simulink model "polydome_python"  (R2020b)
settings: Solver=VariableStepAuto  StartTime=0.0  StopTime=365 * 24 * 3600  RelTol=1e-3
model workspace: external: MAT-File /home/radu/Projects/Master-Project/Simulink/polydome_params.mat (data not in the file)
values from neighbouring files (symbols this model uses):
  Tsample = 900    [model_identification.m]
  window_roof_size = [5 5]    [main.m]
undefined symbols (not defined in the file or in its folder): DE_TRY2010_04_averageYear, Dreifach, f, path_carnot, Wärmeschutzglas
libraries: carnot x13, instrumentlib x3, simulink_extras x2
settings Model: PauseTimes=9200  OrderedModelArguments=off  Creator=radu  LastModifiedBy=radu
settings HardwareCC: ProdBitPerLong=64  ProdHWDeviceType=Intel->x86-64 (Linux 64)

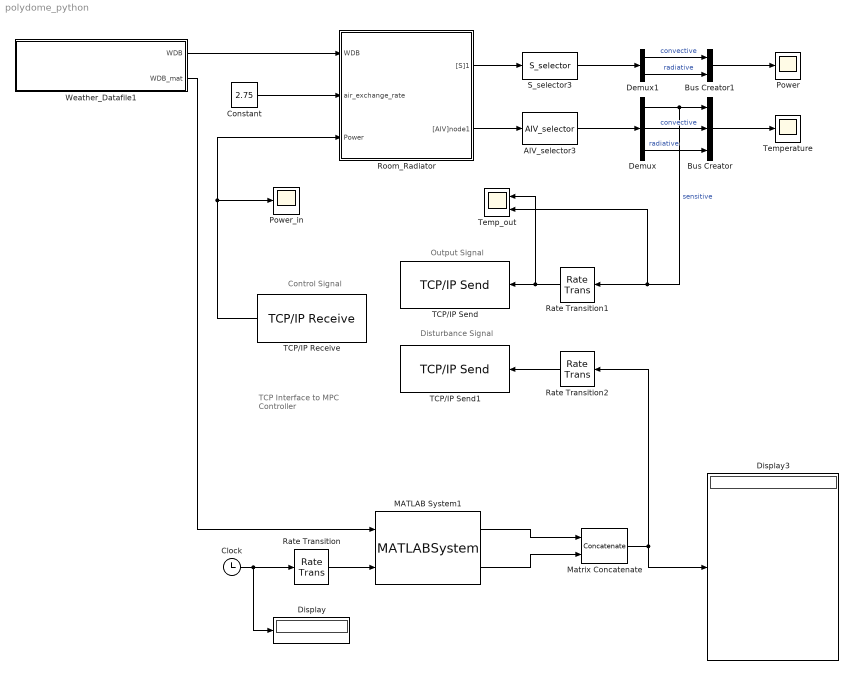
== system polydome_python ==
  note: TCP Interface to
      | MPC Controller
  note: Control Signal
  note: Output Signal
  note: Disturbance Signal
  AIV_selector3 : carnot/Outputs/AIV_selector  e1=on  e2=on  e3=on  e4=off  e5=off  e6=off  e7=off  e8=off  e9=off
      settings: SourceProductName=Carnot
  Bus Creator : BusCreator  Inputs=3
  Bus Creator1 : BusCreator  Inputs=2
  Clock : Clock
  Constant : Constant  Value=2.75
  Demux : Demux  Outputs=3
  Demux1 : Demux  Outputs=2
  Display : Display
  Display3 : Display
  MATLAB System1 : MATLABSystem  System=weather_predictor  TimeStep=Tsample  N=8  SimulateUsing=Interpreted execution
      mask Type: weather_predictor
      mask Display:
      | disp('weather_predictor');
      | port_label('input',1,'wdb_mat');
      | port_label('input',2,'timestamp');
      | port_label('output',1,'w');
      | port_label('output',2,'w_hat');
  Matrix Concatenate : Concatenate  Mode=Multidimensional array
  Power : Scope
  Power_in : Scope
  Rate Transition : RateTransition  OutPortSampleTime=Tsample
  Rate Transition1 : RateTransition  OutPortSampleTime=Tsample
  Rate Transition2 : RateTransition  OutPortSampleTime=Tsample
  Room_Radiator : Subsystem  AncestorBlock=carnot/Load/Houses/Room_Radiator  mask(room){t0=23, temp_neighbour=12}
      mask prompts: t0 "start temperature of rooms in °C"; temp_neighbour "temperature of rooms above and below in °C"
      mask help:
      | The block models of a heat transfer characteristic of two neighbour rooms.
      | Use "look under mask" to set up the models parameters (initial conditions,
      | floors and wall characteristics...)
      mask init:
      | AIV_neighbour = [0 temp_neighbour temp_neighbour 0 0 0 0 0 0];
      | zonefloordist2grnd = 0;
      mask Help: web(fullfile(path_carnot('help'),'Room_Radiator.html'),'-helpbrowser')
      mask Display: plot(0,0,100,100,[30,30,60,60,30],[20,50,50,20,20],[47,47,56,56,47],[40,30,30,40,40],[42,42,34,34],[20,40,40,20],[62,45,28],[48,70,48])
  S_selector3 : carnot/Outputs/S_selector  e1=off  e2=off  e3=off  e4=off  e5=off  e6=off  e7=on  e8=on  e9=off  e10=off  e11=off  e12=off  e13=off
      settings: SourceProductName=Carnot
  TCP/IP Receive : instrumentlib/TCP//IP Receive  Host=127.0.0.1  Port=10001  DataSize=[1 1]  EnableBlockingMode=on  Timeout=100  SampleTime=Tsample  DataType=double  ByteOrder=BigEndian  ASCIIFormatting=%f,  Terminator=LF
  TCP/IP Send : instrumentlib/TCP//IP Send  Host=127.0.0.1  Port=10000  EnableBlockingMode=on  Timeout=10  ByteOrder=BigEndian  TransferDelay=on
  TCP/IP Send1 : instrumentlib/TCP//IP Send  Host=127.0.0.1  Port=10002  EnableBlockingMode=on  Timeout=10  ByteOrder=BigEndian  TransferDelay=on
  Temp_out : Scope  NumInputPorts=2
  Temperature : Scope
  Weather_Datafile1 : Subsystem  AncestorBlock=carnot/Weather/Weather_Datafile  mask(Weather Datafile){PathName=path_carnot('data'), FileName='DE_TRY2010_12_averageYear.mat', UserParam=off, VariableName=DE_TRY2010_04_averageYear, SampleTime=3600}
      mask prompts: PathName "Selected path"; FileName "File"; UserParam "Edit file and path"; VariableName "Simulink:blkprm_prompts:FromWksData"; SampleTime "Timestep in data"
      mask help:
      | Loads weather data in a variable in the mask workspace and extends it according to the simulation interval. A "From Workspace" block in the subsystem uses this variable. The file must contain data in the weather data format of Carnot (type "help WDB_format" in Command window). A Unit-Delay with the timestep of the data forces the model to a maximum timestep equal to the data timestep. This "Timestep in data" is shown as information in the "Selection" frame.
      | Use of buttons in the "Picking a file" frame:
      | 1) "From selected path" opens a window to chose a data file from the "Selected path" shown in the "Selection" frame.
      | 2) "Carnot public data" opens a window to chose a data file from the public data folder in Carnot. The "Path" is set to the public data folder.
      | 3) "Carnot internal data" opens a window to chose a data file from the internal data folder in Carnot. The "Path" is set to the internal data folder.
      | "File" shows the name of the selected file, "Path" the folder where it is located. You can allow editing "File" and "Path" with the checkbox. Be aware that the buttons in the "Picking a file" frame will anyway overwrite the edited values.
      mask init:
      | [ok,VariableName] = CarnotCallbacks_Data_from_File('LoadData', ...
      |     gcbh, PathName, FileName);
      mask Help: web(fullfile(path_carnot('help'),'WeatherDatafile.html'),'-helpbrowser')
      mask Callback UserParam: ok = CarnotCallbacks_Data_from_File('UserMaskEnable',gcbh);
      mask TypeOptions VariableName: FromWorkspace/VariableName
      mask TypeOptions SampleTime: UnitDelay/SampleTime
      mask DialogControl ParameterGroupVar Prompt: Picking a file
      mask DialogControl Control2 Prompt: From selected path
      mask DialogControl Control2 Callback: ok = CarnotCallbacks_Data_from_File('GetFilename',gcbh, 'selected');
      mask DialogControl Control3 Prompt: Carnot public data
      mask DialogControl Control3 Callback: ok = CarnotCallbacks_Data_from_File('GetFilename',gcbh, 'public');
      mask DialogControl Control4 Prompt: Carnot internal data
      mask DialogControl Control4 Callback: ok = CarnotCallbacks_Data_from_File('GetFilename',gcbh, 'internal');
      mask DialogControl Container3 Prompt: Chosen file
      mask DialogControl VariableName Prompt: Data:
      mask Display: disp(['Weather data file:\n', FileName(1:end-4)])
  wires:
  S_selector3/1 -> Demux1/1
  Demux1/1 -> Bus Creator1/1  "convective"
  Demux1/2 -> Bus Creator1/2  "radiative"
  AIV_selector3/1 -> Demux/1
  Room_Radiator/2("[AIV]node1") -> AIV_selector3/1
  Bus Creator1/1 -> Power/1
  Weather_Datafile1/1(WDB) -> Room_Radiator/1(WDB)
  Demux/2 -> Bus Creator/2  "convective"
  Constant/1 -> Room_Radiator/2(air_exchange_rate)
  Demux/3 -> Bus Creator/3  "radiative"
  Bus Creator/1 -> Temperature/1
  Demux/1 -> Bus Creator/1, Temp_out/2, Rate Transition1/1  "sensitive"
  Room_Radiator/1("[S]1") -> S_selector3/1
  Clock/1 -> Rate Transition/1, Display/1
  Weather_Datafile1/2(WDB_mat) -> MATLAB System1/1
  Rate Transition/1 -> MATLAB System1/2
  TCP/IP Receive/1 -> Room_Radiator/3(Power), Power_in/1
  Rate Transition1/1 -> Temp_out/1, TCP/IP Send/1
  Rate Transition2/1 -> TCP/IP Send1/1
  MATLAB System1/1 -> Matrix Concatenate/1
  MATLAB System1/2 -> Matrix Concatenate/2
  Matrix Concatenate/1 -> Rate Transition2/1, Display3/1

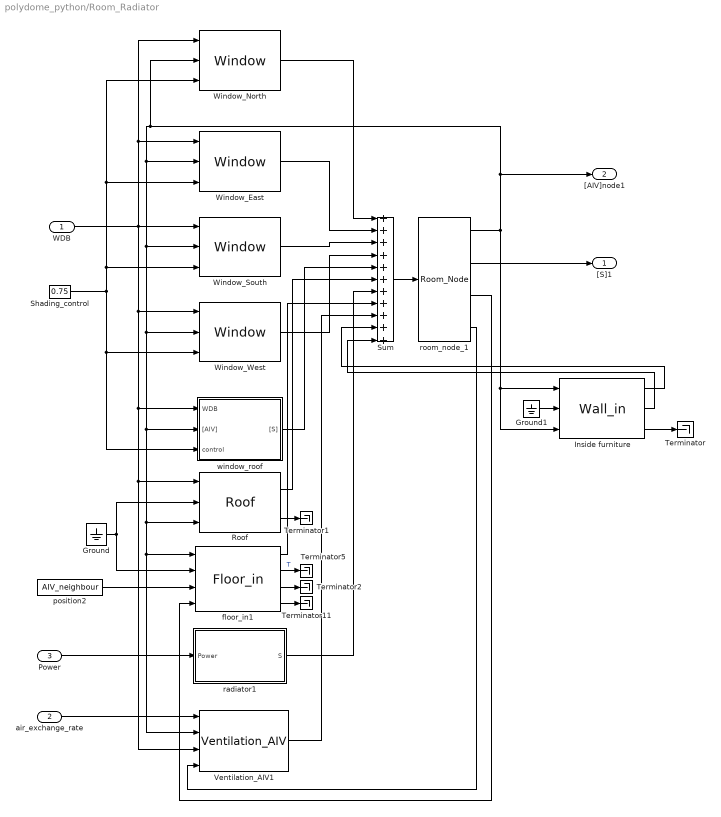
== system polydome_python/Room_Radiator ==
  WDB : Inport
  air_exchange_rate : Inport  Port=2
  Power : Inport  Port=3
  Ground : Ground
  Ground1 : Ground
  Inside furniture : carnot/Basic/Thermal_Models/Wall_in  wallsize=(0.25)*[25 25]*1.8*(1/2)  d=[0.04]  cond=[0.3]  cwall=[1400]  rho=[600]*2  emission_in=.96  dactive=[-1]  t0=t0  tau=10*3600
      settings: SourceProductName=Carnot
  Roof : carnot/Basic/Thermal_Models/Roof  wallsize=wall_size  pos=roof_position  t0=t0  d=node_thickness  cond=node_conductivity  cwall=node_capacity  rho=node_density  reflectground=0.2  abs_emiss=[0.6, 0.9, 0.9]  tau=1000*3600  dactive=-1
      settings: SourceProductName=Carnot
  Shading_control : Constant  Value=0.75
  Sum : Sum  Inputs=11  InputSameDT=on  SaturateOnIntegerOverflow=on  OutDataTypeStr=Inherit: Same as first input
  Terminator{,1..2,5,11} (5 alike) : Terminator
  Ventilation_AIV1 : carnot/Source/Ventilation/Ventilation_AIV  co2=400
      settings: SourceProductName=Carnot
  Window_East : carnot/Basic/Thermal_Models/Window  pos=-80  windowsize=window_size  frame=surface_part  Ug=U  gvalue=g  tauzero=v_g  numpanes=2  d=[0.004 0.004]  rho=[2500 2500]  cp="[1008  1008]"  t0=t0  misc=[0.2 0.1 1 1]  shad_type=Exterior Screen  type_glazing=Dreifach-Wärmeschutzglas  tau_shad=0.01  bli_a=0.05  bli_b=1  bli_c=0.05  bli_d=0.05  bli_alpha=90  bli_refl=0.2
      settings: SourceProductName=Carnot
  Window_North : carnot/Basic/Thermal_Models/Window  pos=-170  windowsize=window_size  frame=surface_part  Ug=U  gvalue=g  tauzero=v_g  numpanes=2  d=[0.004 0.004]  rho=[2500 2500]  cp="[1008  1008]"  t0=t0  misc=[0.2 0.1 1 1]  shad_type=Exterior Screen  type_glazing=Dreifach-Wärmeschutzglas  tau_shad=0.01  bli_a=0.05  bli_b=1  bli_c=0.05  bli_d=0.05  bli_alpha=90  bli_refl=0.2
      settings: SourceProductName=Carnot
  Window_South : carnot/Basic/Thermal_Models/Window  pos=10  windowsize=window_size  frame=surface_part  Ug=U  gvalue=g  tauzero=v_g  numpanes=2  d=[0.004 0.004]  rho=[2500 2500]  cp="[1008  1008]"  t0=t0  misc=[0.2 0.1 1 1]  shad_type=Exterior Screen  type_glazing=Dreifach-Wärmeschutzglas  tau_shad=0.01  bli_a=0.05  bli_b=1  bli_c=0.05  bli_d=0.05  bli_alpha=90  bli_refl=0.2
      settings: SourceProductName=Carnot
  Window_West : carnot/Basic/Thermal_Models/Window  pos=100  windowsize=window_size  frame=surface_part  Ug=U  gvalue=g  tauzero=v_g  numpanes=2  d=[0.004 0.004]  rho=[2500 2500]  cp="[1008  1008]"  t0=t0  misc=[0.2 0.1 1 1]  shad_type=Exterior Screen  type_glazing=Dreifach-Wärmeschutzglas  tau_shad=0.01  bli_a=0.05  bli_b=1  bli_c=0.05  bli_d=0.05  bli_alpha=90  bli_refl=0.2
      settings: SourceProductName=Carnot
  floor_in1 : carnot/Basic/Thermal_Models/Floor_in  wallsize=ceiling_size  t0=t0  d=layer_thickness  cond=layer_conductivity  cwall=layer_capacity  rho=layer_density  misc=[0.9 0.9]  dactive=-1  tau=1000*3600
      settings: SourceProductName=Carnot
  position2 : Constant  Value=AIV_neighbour
  radiator1 : Subsystem  AncestorBlock=carnot/Source/Heat_Exchanger/Radiator_AIV  mask(radiator){pnom=500, dtnom=40, expo=1.3, mcap=5*4182, ra=0.47, tini=24, lin=0, qua=1000}
      mask prompts: pnom "nominal power per unit in W"; dtnom "nominal temperature difference in K"; expo "radiator exponent (> 0)"; mcap "mass * capacity per unit in J/K"; ra "radiative part of heat transfer (0..1)"; tini "initial temperature in degree Celsius"; lin "linear pressure drop dependace of massflow in Pa*s/kg"; qua "quadratic pressure drop dependace of massflow in Pa*s²/kg²"
      mask help: Calculates the power of a radiator according to the nominal power the and the temperaure difference.
      mask init:
      | ra = max(0, min(1, ra));
      | co = 1-ra;
      mask Help: web(['file:///' fullfile(path_carnot('help'),'Radiator.html')],'-helpbrowser')
      mask DialogControl ParameterTabVar0 Prompt: Thermal
      mask DialogControl ParameterTabVar01 Prompt: Hydraulic
      mask Display: plot(-20,0,120,90,[20 90 90 20 20],[20 20 70 70 20],[30 30],[25 65],[40 40],[25 65],[50 50],[25 65],[60 60],[25 65],[70 70],[25 65],[80 80],[25 65],[15 20],[25 25],[15 20],[65 65])
  room_node_1 : carnot/Basic/Thermal_Models/Room_Node  zoneairvolume=25*25*5  zoneheight=2.5  zonestartTEMP=t0  zonestartWATER=55  timeconst=100  heatperfect=natural  lookuptime=[0 24]*3600  lookupvalue=[20 20]  AirPressure=101300  calc_p=off
      settings: SourceProductName=Carnot
  window_roof : Subsystem  AncestorBlock=carnot/Basic/Thermal_Models/Window  mask(window){pos=0, windowsize=window_roof_size, frame=0.1, Ug=1.8, gvalue=0.7, tauzero=0.8, numpanes=2, d=[0.004 0.004], rho=[2500 2500], cp=[1008  1008], t0=t0, misc=[0.2 0.1 1 1], shad_type=No shading, type_glazing=Dreifach-Wärmeschutzglas, tau_shad=0.01, bli_a=0.05, bli_b=1, bli_c=0.05, bli_d=0.05, bli_alpha=90, bli_refl=0.2}
      mask prompts: pos "azimut (0=south, east = -90)"; windowsize "size of window [m] [height width]"; frame "part of frame of the surface (0..1)"; Ug "heat transfer coefficient (U-value) [W/m²K]"; gvalue "total solar energy transmittance (g-value) [0..1]"; tauzero "transmittance in visible range of the sunlight [0..1]"; numpanes "number of glass panes [1..4]"; d "thickness of glass panes [m] (vector with one element per pane)"; rho "density of glass [kg/m³] (vector with one element per pane)"; cp "capacity of glass [J/(kg*K)] (vector with one element per pane)"; t0 "initial temperature [°C]"; misc "[reflection_ground absorption_out emission_out emission_in]"; shad_type "shading type [no Shading/exterior/interior]"; type_glazing "glazing type"; tau_shad "solar transmittance of shading element [0..1]"; bli_a "a  Depth of blind blades [m]"; bli_b "b heigth of blind blades [m]"; bli_c "c distance of "b" to back end of blind blade [m]"; bli_d "d offset between blind blades [m]"; bli_alpha "blind angle  (0=closed, 90=horizontal) [0..90]"; bli_refl "optical reflectance of blind surface [0..1]"
      mask help:
      | The window model evaluates the g-value, the total energy transmission tau and the u-value to build up a two node model.
      | control input [0..1] = fraction of shading (0 - no shading,   1 - full shading)
      mask init:
      | % Geometry
      | h = windowsize(1);
      | w = windowsize(2);
      | windowsurface = h*w;
      | if length(pos) == 1
      |     pos = [0  pos 0]; % pos is [inclination azimut rotation]
      | end
      | 
      | % Optics
      | reflectground = max(0, min(1, misc(1)));
      | absorption_out = max(0, min(1, misc(2)));
      | emission_out = max(0, min(1, misc(3)));
      | emission_in = max(0, min(1, misc(4)));
      | 
      | % Thermal
      | R_norm_in = 1/8;     % h_int = 8 W/m²/K set according to ISO
      | R_norm_out = 1/25;   % h_out = 25 W/m²/K set according to ISO
      | Rwin = 1/Ug - R_norm_in - R_norm_out;
      | % C = sum(cp.*rho.*d.^2); % old equation
      | C = sum(cp.*rho.*d); % corrected equation, hf 29nov2017
      | timeconst = Rwin*C/2;
      mask Help: web(fullfile(path_carnot('help'),'WindowWithShading.html'),'-helpbrowser')
      mask TypeOptions shad_type: No shading | Exterior Screen | Interior Screen | Venetian Blind
      mask Callback shad_type:
      | switch get_param(gcb,'shad_type')
      |         case 'No shading' % nr. 1 no shading
      |             set_param(gcb,'MaskVisibilities',{'on','on','on','on','on','on','on','on','on','on','on','on','on','off','off','off','off','off','off','off','off'});
      |         case 'Exterior Screen' % nr. 2 external screen
      |             set_param(gcb,'MaskVisibilities',{'on','on','on','on','on','on','on','on','on','on','on','on','on','off','on','off','off','off','off','off','off'});
      |         case 'Interior Screen' % nr. 3 Interior Screen
      |             set_param(gcb,'MaskVisibilities',{'on','on','on','on','on','on','on','on','on','on','on','on','on','on','on','off','off','off','off','off','off'});
      |         case 'Venetian Blind' % nr. 4 venetian blind
      |             set_param(gcb,'MaskVisibilities',{'on','on','on','on','on','on','on','on','on','on','on','on','on','off','off','on','on','on','on','on','on'});
      |     end
      mask TypeOptions type_glazing: Zweifachglas normal | Zweifach-Wärmeschutzglas | Zweifach-Kombiglas 73/41 | Zweifach-Kombiglas 50/24 | Dreifachglas normal | Dreifach-Wärmeschutzglas
  "[S]1" : Outport  VectorParamsAs1DForOutWhenUnconnected=off
  "[AIV]node1" : Outport  Port=2  VectorParamsAs1DForOutWhenUnconnected=off
  wires:
  floor_in1/4 -> Terminator11/1
  room_node_1/2 -> "[S]1"/1
  floor_in1/3 -> Terminator2/1
  floor_in1/1 -> Sum/8
  Ventilation_AIV1/1 -> Sum/9
  room_node_1/4 -> Ventilation_AIV1/4
  room_node_1/3 -> floor_in1/4
  position2/1 -> floor_in1/3
  air_exchange_rate/1 -> Ventilation_AIV1/1
  room_node_1/1 -> Inside furniture/3, Inside furniture/1, Window_North/2, Window_East/2, Window_South/2, window_roof/2("[AIV]"), floor_in1/1, Ventilation_AIV1/2, Roof/3, Window_West/2, "[AIV]node1"/1
  floor_in1/2 -> Terminator5/1  "T"
  Sum/1 -> room_node_1/1
  WDB/1 -> Window_South/1, Window_East/1, Window_North/1, Window_West/1, window_roof/1(WDB), Roof/1, Ventilation_AIV1/3
  Ground/1 -> floor_in1/2, Roof/2
  radiator1/1(S) -> Sum/7
  Roof/1 -> Sum/6
  window_roof/1("[S]") -> Sum/5
  Window_West/1 -> Sum/4
  Window_South/1 -> Sum/3
  Window_East/1 -> Sum/2
  Window_North/1 -> Sum/1
  Roof/2 -> Terminator1/1
  Power/1 -> radiator1/1(Power)
  Shading_control/1 -> window_roof/3(control), Window_West/3, Window_South/3, Window_East/3, Window_North/3
  Inside furniture/1 -> Sum/10
  Inside furniture/2 -> Sum/11
  Ground1/1 -> Inside furniture/2
  Inside furniture/3 -> Terminator/1

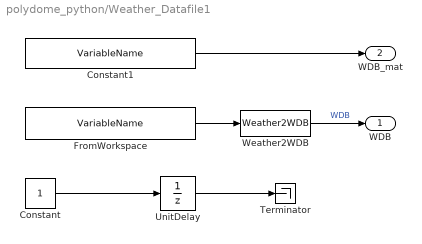
== system polydome_python/Weather_Datafile1 ==
  Constant : Constant
  Constant1 : Constant  Value=VariableName  SampleTime=-1
  FromWorkspace : FromWorkspace  VariableName=VariableName  SampleTime=-1  ZeroCross=off  OutputAfterFinalValue=Holding final value
  Terminator : Terminator
  UnitDelay : UnitDelay  SampleTime=SampleTime  HasFrameUpgradeWarning=on
  Weather2WDB : carnot/Toolbox/Weather2WDB
      settings: SourceProductName=Carnot
  WDB : Outport  VectorParamsAs1DForOutWhenUnconnected=off
  WDB_mat : Outport  Port=2
  wires:
  UnitDelay/1 -> Terminator/1
  Constant/1 -> UnitDelay/1
  FromWorkspace/1 -> Weather2WDB/1
  Weather2WDB/1 -> WDB/1  "WDB"
  Constant1/1 -> WDB_mat/1

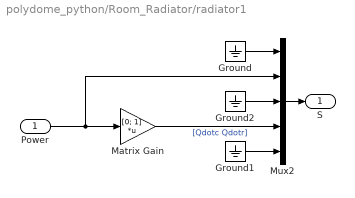
== system polydome_python/Room_Radiator/radiator1 ==
  Power : Inport
  Ground : Ground
  Ground1 : Ground
  Ground2 : Ground
  Matrix Gain : Gain  Gain=[0; 1]  Multiplication=Matrix(K*u)  SaturateOnIntegerOverflow=on  OutDataTypeStr=Inherit: Same as input  ParamDataTypeStr=Inherit: Same as input
  Mux2 : Mux  Inputs=[4 1 1 2 5]
  S : Outport  VectorParamsAs1DForOutWhenUnconnected=off
  wires:
  Power/1 -> Mux2/2, Matrix Gain/1
  Matrix Gain/1 -> Mux2/4  "[Qdotc Qdotr]"
  Mux2/1 -> S/1
  Ground1/1 -> Mux2/5
  Ground2/1 -> Mux2/3
  Ground/1 -> Mux2/1

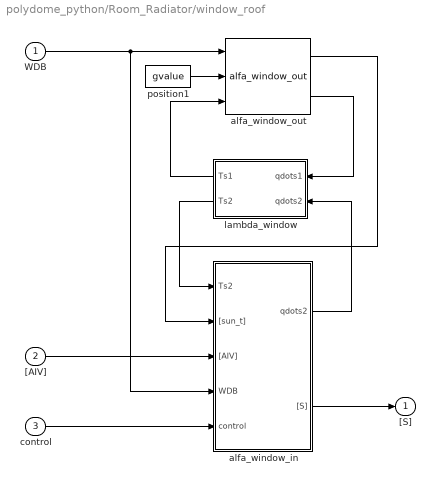
== system polydome_python/Room_Radiator/window_roof ==
  WDB : Inport
  "[AIV]" : Inport  Port=2
  control : Inport  Port=3
  alfa_window_in : Subsystem  mask(ALFA){}
      mask help:
      | Convective and radiative heat transfer at the INDOOR SURFACE OF A VERTICAL WINDOW with 1-4 layers (each 3 ... 8 mm thick).
      |
      | Ts  : temperature of window surface, °C,
      | [sun_t]  : sun data (incidence angle, direct and diffuse radiation
      |     at tilted window surface),
      | [AIV]  : conditions of zone node,
      | qdots  : specific heat flow into window construction, W/m^2,
      | [S]  : heat and air flow to zone node.
  alfa_window_out : carnot/Basic/Heat_Transfer/alfa_window_out  pos=pos  absorption_out=absorption_out  emission_out=emission_out  frame=frame
      settings: SourceProductName=Carnot
  lambda_window : Subsystem  mask(LAMBDA){}
      mask help:
      | Heat conduction through a transparent component (window).
      |
      | qdots1	: specific heat flow vertical on surface 1, W/m²
      | qdots2	: specific heat flow vertical on surface 2, W/m²
      | Ts1	: temperature of surface 1, °C
      | Ts2	: temperature of surface 2, °C
      |
      | NOTE CONVENTION for INPUT NUMBER:
      | "1"	  indoor surface of an outer window OR
      | 	  surface "a" of an inner window OR
      |  	  surface "f" of a glass floor
      |
      | "2"	  outdoor surface of a window OR
      | 	  surface "b" of an inner window OR
      |  	  surface "c" of a glass ceiling
  position1 : Constant  Value=gvalue
  "[S]" : Outport  VectorParamsAs1DForOutWhenUnconnected=off
  wires:
  lambda_window/1(Ts1) -> alfa_window_out/3
  WDB/1 -> alfa_window_out/1, alfa_window_in/4(WDB)
  "[AIV]"/1 -> alfa_window_in/3("[AIV]")
  alfa_window_in/1(qdots2) -> lambda_window/2(qdots2)
  alfa_window_in/2("[S]") -> "[S]"/1
  lambda_window/2(Ts2) -> alfa_window_in/1(Ts2)
  alfa_window_out/2 -> lambda_window/1(qdots1)
  alfa_window_out/1 -> alfa_window_in/2("[sun_t]")
  control/1 -> alfa_window_in/5(control)
  position1/1 -> alfa_window_out/2

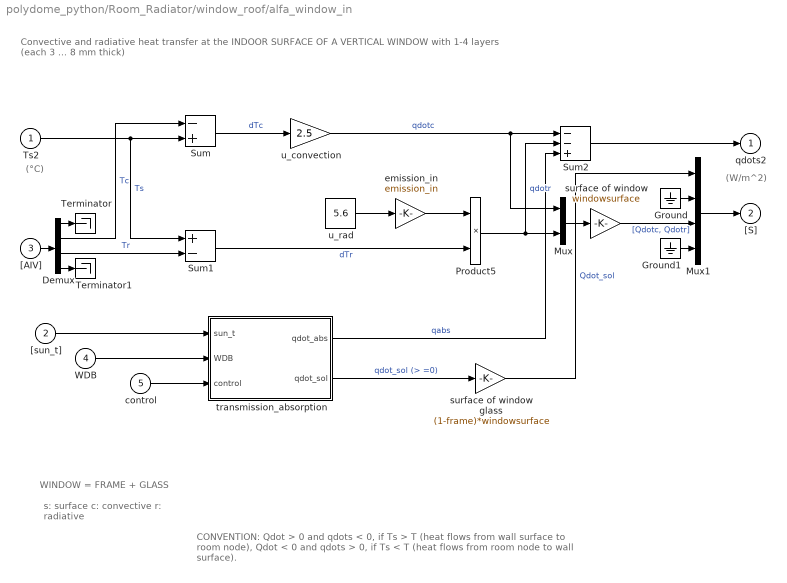
== system polydome_python/Room_Radiator/window_roof/alfa_window_in ==
  note: (W/m^2)
  note: CONVENTION:
      | Qdot > 0 and qdots < 0, if Ts > T (heat flows from wall surface to room node),
      | Qdot < 0 and qdots > 0, if Ts < T (heat flows from room node to wall surface).
  note: s: surface
      | c: convective
      | r: radiative
  note: WINDOW = FRAME + GLASS
  note: Convective and radiative heat transfer at the INDOOR SURFACE OF A VERTICAL WINDOW
      | with 1-4 layers (each 3 ... 8 mm thick)
  note: (°C)
  Ts2 : Inport
  "[sun_t]" : Inport  Port=2
  "[AIV]" : Inport  Port=3
  WDB : Inport  Port=4
  control : Inport  Port=5
  Demux : Demux  Outputs=[1 1 1 6]
      settings: DisplayOption=none
  Ground : Ground
  Ground1 : Ground
  Mux : Mux  Inputs=2
  Mux1 : Mux  Inputs=[1 5 2 5]
  Product5 : Product  InputSameDT=on  RndMeth=Zero  SaturateOnIntegerOverflow=on  OutDataTypeStr=Inherit: Same as first input
  Sum : Sum  Inputs=-+  InputSameDT=on  SaturateOnIntegerOverflow=on  OutDataTypeStr=Inherit: Same as first input
  Sum1 : Sum  Inputs=+-  InputSameDT=on  SaturateOnIntegerOverflow=on  OutDataTypeStr=Inherit: Same as first input
  Sum2 : Sum  Inputs=--+  InputSameDT=on  SaturateOnIntegerOverflow=on  OutDataTypeStr=Inherit: Same as first input
  Terminator : Terminator
  Terminator1 : Terminator
  emission_in : Gain  Gain=emission_in  SaturateOnIntegerOverflow=on  OutDataTypeStr=Inherit: Same as input  ParamDataTypeStr=Inherit: Same as input
  surface of window : Gain  Gain=windowsurface  SaturateOnIntegerOverflow=on  OutDataTypeStr=Inherit: Same as input  ParamDataTypeStr=Inherit: Same as input
  surface of window glass : Gain  Gain=(1-frame)*windowsurface  SaturateOnIntegerOverflow=on  OutDataTypeStr=Inherit: Same as input  ParamDataTypeStr=Inherit: Same as input
  transmission_absorption : Subsystem
  u_convection : Gain  Gain=2.5  SaturateOnIntegerOverflow=on  OutDataTypeStr=Inherit: Same as input  ParamDataTypeStr=Inherit: Same as input
  u_rad : Constant  Value=5.6
  qdots2 : Outport  VectorParamsAs1DForOutWhenUnconnected=off
  "[S]" : Outport  Port=2  VectorParamsAs1DForOutWhenUnconnected=off
  wires:
  Ground1/1 -> Mux1/4
  Ground/1 -> Mux1/2
  Mux1/1 -> "[S]"/1
  Sum2/1 -> qdots2/1
  Demux/4 -> Terminator1/1
  "[AIV]"/1 -> Demux/1
  Demux/1 -> Terminator/1
  Mux/1 -> surface of window/1
  emission_in/1 -> Product5/1
  Sum1/1 -> Product5/2  "dTr"
  u_rad/1 -> emission_in/1
  Ts2/1 -> Sum/2, Sum1/1  "Ts"
  Product5/1 -> Mux/2, Sum2/2  "qdotr"
  u_convection/1 -> Sum2/1, Mux/1  "qdotc"
  "[sun_t]"/1 -> transmission_absorption/1(sun_t)
  surface of window glass/1 -> Mux1/1  "Qdot_sol"
  surface of window/1 -> Mux1/3  "[Qdotc, Qdotr]"
  Demux/2 -> Sum/1  "Tc"
  Sum/1 -> u_convection/1  "dTc"
  Demux/3 -> Sum1/2  "Tr"
  transmission_absorption/2(qdot_sol) -> surface of window glass/1  "qdot_sol (> =0)"
  transmission_absorption/1(qdot_abs) -> Sum2/3  "qabs"
  WDB/1 -> transmission_absorption/2(WDB)
  control/1 -> transmission_absorption/3(control)

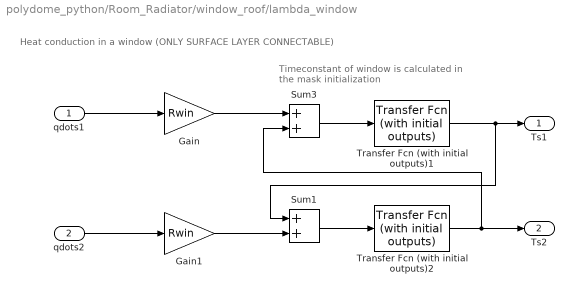
== system polydome_python/Room_Radiator/window_roof/lambda_window ==
  note: Timeconstant of window is calculated
      | in the mask initialization
  note: Heat conduction in a window (ONLY SURFACE LAYER CONNECTABLE)
  qdots1 : Inport
  qdots2 : Inport  Port=2
  Gain : Gain  Gain=Rwin
  Gain1 : Gain  Gain=Rwin
  Sum1 : Sum  InputSameDT=on  SaturateOnIntegerOverflow=on  OutDataTypeStr=Inherit: Same as first input
  Sum3 : Sum  InputSameDT=on  SaturateOnIntegerOverflow=on  OutDataTypeStr=Inherit: Same as first input
  Transfer Fcn (with initial outputs)1 : simulink_extras/Additional Linear/Transfer Fcn (with initial outputs)  N=[1]  D=[timeconst 1]  Y0=t0  U0=t0
  Transfer Fcn (with initial outputs)2 : simulink_extras/Additional Linear/Transfer Fcn (with initial outputs)  N=[1]  D=[timeconst 1]  Y0=t0  U0=t0
  Ts1 : Outport  VectorParamsAs1DForOutWhenUnconnected=off
  Ts2 : Outport  Port=2  VectorParamsAs1DForOutWhenUnconnected=off
  wires:
  Gain1/1 -> Sum1/2
  Gain/1 -> Sum3/1
  Sum1/1 -> Transfer Fcn (with initial outputs)2/1
  qdots2/1 -> Gain1/1
  Sum3/1 -> Transfer Fcn (with initial outputs)1/1
  qdots1/1 -> Gain/1
  Transfer Fcn (with initial outputs)1/1 -> Ts1/1, Sum1/1
  Transfer Fcn (with initial outputs)2/1 -> Sum3/2, Ts2/1

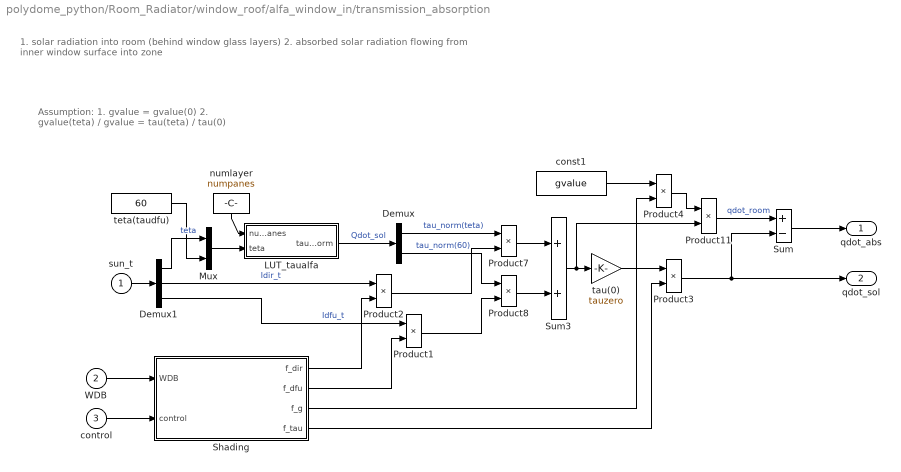
== system polydome_python/Room_Radiator/window_roof/alfa_window_in/transmission_absorption ==
  note: 1. solar radiation into room (behind window glass layers)
      | 2. absorbed solar radiation flowing from inner window surface into zone
  note: Assumption:
      | 1. gvalue = gvalue(0)
      | 2. gvalue(teta) / gvalue = tau(teta) / tau(0)
  sun_t : Inport
  WDB : Inport  Port=2
  control : Inport  Port=3
  Demux : Demux  Outputs=2
      settings: DisplayOption=none
  Demux1 : Demux  Outputs=3
      settings: DisplayOption=none
  LUT_taualfa : Subsystem  mask(LOOK UP TABLE){}
      mask help:
      | Normalized RADIATION TRANSMISSION COEFFICIENT of a window glass layer stack with 1, 2, 3 or 4 layers depending on the incidence angle.
      |
      | teta		: incidence angle = angle between surface normal and
      | 	                incidence direction, degree
      | numlayer	: number of layers within the window glass, [1,4].
      | tau		: transmission of glass layer stack, [0,1]
      |
      | NOTE: This block is defined for pane thickness between 3 and 6 mm.
  Mux : Mux  Inputs=2
  Product{1..4,7..8} (6 alike) : Product  InputSameDT=on  RndMeth=Zero  SaturateOnIntegerOverflow=on  OutDataTypeStr=Inherit: Same as first input
  Product11 : Product  Inputs=**  InputSameDT=on  RndMeth=Zero  SaturateOnIntegerOverflow=on  OutDataTypeStr=Inherit: Same as first input
  Shading : Subsystem
  Sum : Sum  Inputs=+-  InputSameDT=on  SaturateOnIntegerOverflow=on  OutDataTypeStr=Inherit: Same as first input
  Sum3 : Sum  InputSameDT=on  SaturateOnIntegerOverflow=on  OutDataTypeStr=Inherit: Same as first input
  const1 : Constant  Value=gvalue
  numlayer : Constant  Value=numpanes
  tau(0) : Gain  Gain=tauzero  SaturateOnIntegerOverflow=on  OutDataTypeStr=Inherit: Same as input  ParamDataTypeStr=Inherit: Same as input
  teta(taudfu) : Constant  Value=60
  qdot_abs : Outport  VectorParamsAs1DForOutWhenUnconnected=off
  qdot_sol : Outport  Port=2  VectorParamsAs1DForOutWhenUnconnected=off
  wires:
  Mux/1 -> LUT_taualfa/2(teta)
  numlayer/1 -> LUT_taualfa/1(numlpanes)
  teta(taudfu)/1 -> Mux/2
  Demux1/1 -> Mux/1  "teta"
  Sum/1 -> qdot_abs/1
  Product11/1 -> Sum/1  "qdot_room"
  Demux/2 -> Product8/1  "tau_norm(60)"
  Sum3/1 -> tau(0)/1, Product11/2
  Product8/1 -> Sum3/2
  Product7/1 -> Sum3/1
  Demux/1 -> Product7/1  "tau_norm(teta)"
  LUT_taualfa/1(tau_norm) -> Demux/1  "Qdot_sol"
  sun_t/1 -> Demux1/1
  tau(0)/1 -> Product3/1
  Product3/1 -> Sum/2, qdot_sol/1
  Demux1/3 -> Product1/1  "Idfu_t"
  Product1/1 -> Product8/2
  Demux1/2 -> Product2/1  "Idir_t"
  Product2/1 -> Product7/2
  Shading/1(f_dir) -> Product2/2
  Shading/2(f_dfu) -> Product1/2
  Shading/4(f_tau) -> Product3/2
  Product4/1 -> Product11/1
  const1/1 -> Product4/1
  Shading/3(f_g) -> Product4/2
  WDB/1 -> Shading/1(WDB)
  control/1 -> Shading/2(control)

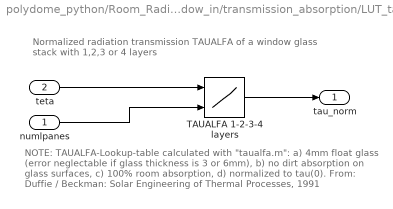
== system polydome_python/Room_Radiator/window_roof/alfa_window_in/transmission_absorption/LUT_taualfa ==
  note: Normalized radiation transmission TAUALFA
      | of a window glass stack with 1,2,3 or 4 layers
  note: NOTE:
      | TAUALFA-Lookup-table calculated with "taualfa.m":
      |   a) 4mm float glass (error neglectable if glass thickness is 3 or 6mm),
      |   b) no dirt absorption on glass surfaces,
      |   c) 100% room absorption,
      |   d) normalized to tau(0).
      |
      | From: Duffie / Beckman: Solar Engineering of Thermal Processes, 1991
  numlpanes : Inport
  teta : Inport  Port=2
  TAUALFA 1-2-3-4 layers : Lookup2D  RowIndex=[0:10:90]  ColumnIndex=[1:4]  Table="[1  1  1  1;.99955 .99912  .9987 .99827;.99787  .9961 .99449 .99298;.99364 .98941 .98618 .98366;.98364 .97519 .97041 .96824;.9601 .94337 .93638 .93624;.90423 .86634 .84734 .84064;.77129 .67843 .61507 .56891;.47436  .3235 .22952 .16682;0  0  0  0]"  SaturateOnIntegerOverflow=on  InputSameDT=on
  tau_norm : Outport  VectorParamsAs1DForOutWhenUnconnected=off
  wires:
  TAUALFA 1-2-3-4 layers/1 -> tau_norm/1
  numlpanes/1 -> TAUALFA 1-2-3-4 layers/2
  teta/1 -> TAUALFA 1-2-3-4 layers/1

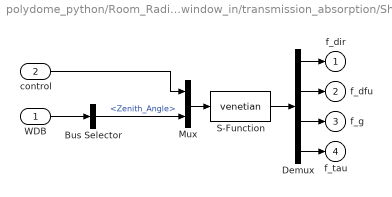
== system polydome_python/Room_Radiator/window_roof/alfa_window_in/transmission_absorption/Shading ==
  WDB : Inport
  control : Inport  Port=2
  Bus Selector : BusSelector  OutputSignals=Zenith_Angle
  Demux : Demux
  Mux : Mux  Inputs=2
  S-Function : S-Function  FunctionName=venetian  Parameters=bli_a, bli_b, bli_c, bli_d, bli_alpha, bli_refl, shad_type, type_glazing, tau_shad  SFunctionDeploymentMode=off  EnableBusSupport=off
  f_dir : Outport  VectorParamsAs1DForOutWhenUnconnected=off
  f_dfu : Outport  Port=2  VectorParamsAs1DForOutWhenUnconnected=off
  f_g : Outport  Port=3  VectorParamsAs1DForOutWhenUnconnected=off
  f_tau : Outport  Port=4  VectorParamsAs1DForOutWhenUnconnected=off
  wires:
  Demux/4 -> f_tau/1
  Demux/3 -> f_g/1
  Demux/2 -> f_dfu/1
  Demux/1 -> f_dir/1
  S-Function/1 -> Demux/1
  Mux/1 -> S-Function/1
  control/1 -> Mux/1
  Bus Selector/1 -> Mux/2  "<Zenith_Angle>"
  WDB/1 -> Bus Selector/1
